simulink model "SWC_HALOUT_type"  (R2021b)
settings: Solver=FixedStepDiscrete  StartTime=0.0  StopTime=10.0  FixedStep=0.005  RelTol=1e-3
undefined symbols (not defined in the file): DIDLen_APPD, DIDLen_APPE, DIDLen_APPPedalZP, DIDLen_APSFunConfig, DIDLen_AutoLock, DIDLen_AutoWipHSpdEN, DIDLen_CALID, DIDLen_CDEODT, DIDLen_CLRDIST, DIDLen_DKCBLESta, DIDLen_DKCKey, DIDLen_DKCSta, DIDLen_DoorNFCAnchorSta, DIDLen_DRLDis, DIDLen_DynoMode, DIDLen_ECUNAME, DIDLen_FDDKCCoordXY, DIDLen_FMHTimer, DIDLen_LFLowPresThre, DIDLen_LFSensorID, DIDLen_LIDAAnchorSta, DIDLen_LRLowPresThre, DIDLen_LRSensorID, DIDLen_MILDIST, DIDLen_NUMPSATRIPSFLTMEMCLR, DIDLen_NVMPedalZP, DIDLen_OBDReq, DIDLen_ODOMETER, DIDLen_PKE, DIDLen_ProtocolId, DIDLen_PSA, DIDLen_QTYPSATRIPS, DIDLen_RFLowPresThre, DIDLen_RFSensorID, DIDLen_RRLowPresThre, DIDLen_RRSensorID, DIDLen_RUNTM, DIDLen_SensorMode, DIDLen_TestGroup, DIDLen_TireSize, DIDLen_TPMSLearnSta, DIDLen_TurnLampFLThreCurr, DIDLen_TurnLampFRThreCurr, DIDLen_TurnLampRLThreCurr, DIDLen_TurnLampRRThreCurr, DIDLen_UIDSta, DIDLen_USSConfig, DIDLen_UWBAnchorSta, DIDLen_VIN, DIDLen_VSS, DIDLen_WhlPres, DIDLen_WhlSensorBattSta, DIDLen_WhlTmp, DIDLen_WipRLSCmdCutFilter, DIDLen_WipRLSCmdHoldFilter, DIDLen_XWDMode, DIDNum_APPD, DIDNum_APPE, DIDNum_APPPedalZP, DIDNum_APSFunConfig ... (+504)
libraries: simulink x893, FVT_lib x320, hdlsllib x6, hcu_lib x5, halout x1
(part 8 of 11)

== system SWC_HALOUT_type/run_SWC_HALOUT_Tx_5ms_sys/OUTP_AFTER/DID_list/uint32Touint8Array49 ==
  In1 : Inport
  Bitwise AND1 : simulink/Logic and Bit Operations/Bitwise Operator  logicop=AND  UseBitMask=on  BitMask=bin2dec('00000000000000000000000011111111')  BitMaskRealWorld=Stored Integer
  Bitwise AND2 : simulink/Logic and Bit Operations/Bitwise Operator  logicop=AND  UseBitMask=on  BitMask=bin2dec('00000000000000001111111100000000')  BitMaskRealWorld=Stored Integer
  Bitwise AND3 : simulink/Logic and Bit Operations/Bitwise Operator  logicop=AND  UseBitMask=on  BitMask=bin2dec('00000000111111110000000000000000')  BitMaskRealWorld=Stored Integer
  Bitwise AND4 : simulink/Logic and Bit Operations/Bitwise Operator  logicop=AND  UseBitMask=on  BitMask=bin2dec('11111111000000000000000000000000')  BitMaskRealWorld=Stored Integer
  Data Type Conversion{1,3..5} (4 alike) : DataTypeConversion  OutDataTypeStr=uint8
  Data Type Conversion2 : DataTypeConversion  OutDataTypeStr=uint32
  Mux2 : Mux
  Shift Arithmetic39 : ArithShift  BitShiftNumber=8  BitShiftDirection=Right
  Shift Arithmetic40 : ArithShift  BitShiftNumber=16  BitShiftDirection=Right
  Shift Arithmetic41 : ArithShift  BitShiftNumber=24  BitShiftDirection=Right
  Out1 : Outport
  wires:
  Bitwise AND4/1 -> Shift Arithmetic41/1
  Bitwise AND1/1 -> Data Type Conversion1/1
  Shift Arithmetic40/1 -> Data Type Conversion4/1
  Shift Arithmetic41/1 -> Data Type Conversion3/1
  Mux2/1 -> Out1/1
  In1/1 -> Data Type Conversion2/1
  Bitwise AND3/1 -> Shift Arithmetic40/1
  Shift Arithmetic39/1 -> Data Type Conversion5/1
  Data Type Conversion3/1 -> Mux2/1
  Bitwise AND2/1 -> Shift Arithmetic39/1
  Data Type Conversion2/1 -> Bitwise AND4/1, Bitwise AND3/1, Bitwise AND1/1, Bitwise AND2/1
  Data Type Conversion5/1 -> Mux2/3
  Data Type Conversion4/1 -> Mux2/2
  Data Type Conversion1/1 -> Mux2/4

== system SWC_HALOUT_type/run_SWC_HALOUT_Tx_5ms_sys/OUTP_AFTER/DID_list/uint32Touint8Array5 ==
  In1 : Inport
  Bitwise AND1 : simulink/Logic and Bit Operations/Bitwise Operator  logicop=AND  UseBitMask=on  BitMask=bin2dec('00000000000000000000000011111111')  BitMaskRealWorld=Stored Integer
  Bitwise AND2 : simulink/Logic and Bit Operations/Bitwise Operator  logicop=AND  UseBitMask=on  BitMask=bin2dec('00000000000000001111111100000000')  BitMaskRealWorld=Stored Integer
  Bitwise AND3 : simulink/Logic and Bit Operations/Bitwise Operator  logicop=AND  UseBitMask=on  BitMask=bin2dec('00000000111111110000000000000000')  BitMaskRealWorld=Stored Integer
  Bitwise AND4 : simulink/Logic and Bit Operations/Bitwise Operator  logicop=AND  UseBitMask=on  BitMask=bin2dec('11111111000000000000000000000000')  BitMaskRealWorld=Stored Integer
  Data Type Conversion{1,3..5} (4 alike) : DataTypeConversion  OutDataTypeStr=uint8
  Data Type Conversion2 : DataTypeConversion  OutDataTypeStr=uint32
  Mux2 : Mux
  Shift Arithmetic39 : ArithShift  BitShiftNumber=8  BitShiftDirection=Right
  Shift Arithmetic40 : ArithShift  BitShiftNumber=16  BitShiftDirection=Right
  Shift Arithmetic41 : ArithShift  BitShiftNumber=24  BitShiftDirection=Right
  Out1 : Outport
  wires:
  Data Type Conversion1/1 -> Mux2/4
  Data Type Conversion4/1 -> Mux2/2
  Data Type Conversion5/1 -> Mux2/3
  Data Type Conversion2/1 -> Bitwise AND2/1, Bitwise AND1/1, Bitwise AND3/1, Bitwise AND4/1
  Bitwise AND2/1 -> Shift Arithmetic39/1
  Data Type Conversion3/1 -> Mux2/1
  Shift Arithmetic39/1 -> Data Type Conversion5/1
  Bitwise AND3/1 -> Shift Arithmetic40/1
  In1/1 -> Data Type Conversion2/1
  Mux2/1 -> Out1/1
  Shift Arithmetic41/1 -> Data Type Conversion3/1
  Shift Arithmetic40/1 -> Data Type Conversion4/1
  Bitwise AND1/1 -> Data Type Conversion1/1
  Bitwise AND4/1 -> Shift Arithmetic41/1

== system SWC_HALOUT_type/run_SWC_HALOUT_Tx_5ms_sys/OUTP_AFTER/DID_list/uint32Touint8Array50 ==
  In1 : Inport
  Bitwise AND1 : simulink/Logic and Bit Operations/Bitwise Operator  logicop=AND  UseBitMask=on  BitMask=bin2dec('00000000000000000000000011111111')  BitMaskRealWorld=Stored Integer
  Bitwise AND2 : simulink/Logic and Bit Operations/Bitwise Operator  logicop=AND  UseBitMask=on  BitMask=bin2dec('00000000000000001111111100000000')  BitMaskRealWorld=Stored Integer
  Bitwise AND3 : simulink/Logic and Bit Operations/Bitwise Operator  logicop=AND  UseBitMask=on  BitMask=bin2dec('00000000111111110000000000000000')  BitMaskRealWorld=Stored Integer
  Bitwise AND4 : simulink/Logic and Bit Operations/Bitwise Operator  logicop=AND  UseBitMask=on  BitMask=bin2dec('11111111000000000000000000000000')  BitMaskRealWorld=Stored Integer
  Data Type Conversion{1,3..5} (4 alike) : DataTypeConversion  OutDataTypeStr=uint8
  Data Type Conversion2 : DataTypeConversion  OutDataTypeStr=uint32
  Mux2 : Mux
  Shift Arithmetic39 : ArithShift  BitShiftNumber=8  BitShiftDirection=Right
  Shift Arithmetic40 : ArithShift  BitShiftNumber=16  BitShiftDirection=Right
  Shift Arithmetic41 : ArithShift  BitShiftNumber=24  BitShiftDirection=Right
  Out1 : Outport
  wires:
  Data Type Conversion1/1 -> Mux2/4
  Data Type Conversion4/1 -> Mux2/2
  Data Type Conversion5/1 -> Mux2/3
  Data Type Conversion2/1 -> Bitwise AND2/1, Bitwise AND1/1, Bitwise AND3/1, Bitwise AND4/1
  Bitwise AND2/1 -> Shift Arithmetic39/1
  Data Type Conversion3/1 -> Mux2/1
  Shift Arithmetic39/1 -> Data Type Conversion5/1
  Bitwise AND3/1 -> Shift Arithmetic40/1
  In1/1 -> Data Type Conversion2/1
  Mux2/1 -> Out1/1
  Shift Arithmetic41/1 -> Data Type Conversion3/1
  Shift Arithmetic40/1 -> Data Type Conversion4/1
  Bitwise AND1/1 -> Data Type Conversion1/1
  Bitwise AND4/1 -> Shift Arithmetic41/1

== system SWC_HALOUT_type/run_SWC_HALOUT_Tx_5ms_sys/OUTP_AFTER/DID_list/uint32Touint8Array51 ==
  In1 : Inport
  Bitwise AND1 : simulink/Logic and Bit Operations/Bitwise Operator  logicop=AND  UseBitMask=on  BitMask=bin2dec('00000000000000000000000011111111')  BitMaskRealWorld=Stored Integer
  Bitwise AND2 : simulink/Logic and Bit Operations/Bitwise Operator  logicop=AND  UseBitMask=on  BitMask=bin2dec('00000000000000001111111100000000')  BitMaskRealWorld=Stored Integer
  Bitwise AND3 : simulink/Logic and Bit Operations/Bitwise Operator  logicop=AND  UseBitMask=on  BitMask=bin2dec('00000000111111110000000000000000')  BitMaskRealWorld=Stored Integer
  Bitwise AND4 : simulink/Logic and Bit Operations/Bitwise Operator  logicop=AND  UseBitMask=on  BitMask=bin2dec('11111111000000000000000000000000')  BitMaskRealWorld=Stored Integer
  Data Type Conversion{1,3..5} (4 alike) : DataTypeConversion  OutDataTypeStr=uint8
  Data Type Conversion2 : DataTypeConversion  OutDataTypeStr=uint32
  Mux2 : Mux
  Shift Arithmetic39 : ArithShift  BitShiftNumber=8  BitShiftDirection=Right
  Shift Arithmetic40 : ArithShift  BitShiftNumber=16  BitShiftDirection=Right
  Shift Arithmetic41 : ArithShift  BitShiftNumber=24  BitShiftDirection=Right
  Out1 : Outport
  wires:
  Bitwise AND4/1 -> Shift Arithmetic41/1
  Bitwise AND1/1 -> Data Type Conversion1/1
  Shift Arithmetic40/1 -> Data Type Conversion4/1
  Shift Arithmetic41/1 -> Data Type Conversion3/1
  Mux2/1 -> Out1/1
  In1/1 -> Data Type Conversion2/1
  Bitwise AND3/1 -> Shift Arithmetic40/1
  Shift Arithmetic39/1 -> Data Type Conversion5/1
  Data Type Conversion3/1 -> Mux2/1
  Bitwise AND2/1 -> Shift Arithmetic39/1
  Data Type Conversion2/1 -> Bitwise AND4/1, Bitwise AND3/1, Bitwise AND1/1, Bitwise AND2/1
  Data Type Conversion5/1 -> Mux2/3
  Data Type Conversion4/1 -> Mux2/2
  Data Type Conversion1/1 -> Mux2/4

== system SWC_HALOUT_type/run_SWC_HALOUT_Tx_5ms_sys/OUTP_AFTER/DID_list/uint32Touint8Array52 ==
  In1 : Inport
  Bitwise AND1 : simulink/Logic and Bit Operations/Bitwise Operator  logicop=AND  UseBitMask=on  BitMask=bin2dec('00000000000000000000000011111111')  BitMaskRealWorld=Stored Integer
  Bitwise AND2 : simulink/Logic and Bit Operations/Bitwise Operator  logicop=AND  UseBitMask=on  BitMask=bin2dec('00000000000000001111111100000000')  BitMaskRealWorld=Stored Integer
  Bitwise AND3 : simulink/Logic and Bit Operations/Bitwise Operator  logicop=AND  UseBitMask=on  BitMask=bin2dec('00000000111111110000000000000000')  BitMaskRealWorld=Stored Integer
  Bitwise AND4 : simulink/Logic and Bit Operations/Bitwise Operator  logicop=AND  UseBitMask=on  BitMask=bin2dec('11111111000000000000000000000000')  BitMaskRealWorld=Stored Integer
  Data Type Conversion{1,3..5} (4 alike) : DataTypeConversion  OutDataTypeStr=uint8
  Data Type Conversion2 : DataTypeConversion  OutDataTypeStr=uint32
  Mux2 : Mux
  Shift Arithmetic39 : ArithShift  BitShiftNumber=8  BitShiftDirection=Right
  Shift Arithmetic40 : ArithShift  BitShiftNumber=16  BitShiftDirection=Right
  Shift Arithmetic41 : ArithShift  BitShiftNumber=24  BitShiftDirection=Right
  Out1 : Outport
  wires:
  Data Type Conversion1/1 -> Mux2/4
  Data Type Conversion4/1 -> Mux2/2
  Data Type Conversion5/1 -> Mux2/3
  Data Type Conversion2/1 -> Bitwise AND2/1, Bitwise AND1/1, Bitwise AND3/1, Bitwise AND4/1
  Bitwise AND2/1 -> Shift Arithmetic39/1
  Data Type Conversion3/1 -> Mux2/1
  Shift Arithmetic39/1 -> Data Type Conversion5/1
  Bitwise AND3/1 -> Shift Arithmetic40/1
  In1/1 -> Data Type Conversion2/1
  Mux2/1 -> Out1/1
  Shift Arithmetic41/1 -> Data Type Conversion3/1
  Shift Arithmetic40/1 -> Data Type Conversion4/1
  Bitwise AND1/1 -> Data Type Conversion1/1
  Bitwise AND4/1 -> Shift Arithmetic41/1

== system SWC_HALOUT_type/run_SWC_HALOUT_Tx_5ms_sys/OUTP_AFTER/DID_list/uint32Touint8Array53 ==
  In1 : Inport
  Bitwise AND1 : simulink/Logic and Bit Operations/Bitwise Operator  logicop=AND  UseBitMask=on  BitMask=bin2dec('00000000000000000000000011111111')  BitMaskRealWorld=Stored Integer
  Bitwise AND2 : simulink/Logic and Bit Operations/Bitwise Operator  logicop=AND  UseBitMask=on  BitMask=bin2dec('00000000000000001111111100000000')  BitMaskRealWorld=Stored Integer
  Bitwise AND3 : simulink/Logic and Bit Operations/Bitwise Operator  logicop=AND  UseBitMask=on  BitMask=bin2dec('00000000111111110000000000000000')  BitMaskRealWorld=Stored Integer
  Bitwise AND4 : simulink/Logic and Bit Operations/Bitwise Operator  logicop=AND  UseBitMask=on  BitMask=bin2dec('11111111000000000000000000000000')  BitMaskRealWorld=Stored Integer
  Data Type Conversion{1,3..5} (4 alike) : DataTypeConversion  OutDataTypeStr=uint8
  Data Type Conversion2 : DataTypeConversion  OutDataTypeStr=uint32
  Mux2 : Mux
  Shift Arithmetic39 : ArithShift  BitShiftNumber=8  BitShiftDirection=Right
  Shift Arithmetic40 : ArithShift  BitShiftNumber=16  BitShiftDirection=Right
  Shift Arithmetic41 : ArithShift  BitShiftNumber=24  BitShiftDirection=Right
  Out1 : Outport
  wires:
  Data Type Conversion1/1 -> Mux2/4
  Data Type Conversion4/1 -> Mux2/2
  Data Type Conversion5/1 -> Mux2/3
  Data Type Conversion2/1 -> Bitwise AND2/1, Bitwise AND1/1, Bitwise AND3/1, Bitwise AND4/1
  Bitwise AND2/1 -> Shift Arithmetic39/1
  Data Type Conversion3/1 -> Mux2/1
  Shift Arithmetic39/1 -> Data Type Conversion5/1
  Bitwise AND3/1 -> Shift Arithmetic40/1
  In1/1 -> Data Type Conversion2/1
  Mux2/1 -> Out1/1
  Shift Arithmetic41/1 -> Data Type Conversion3/1
  Shift Arithmetic40/1 -> Data Type Conversion4/1
  Bitwise AND1/1 -> Data Type Conversion1/1
  Bitwise AND4/1 -> Shift Arithmetic41/1

== system SWC_HALOUT_type/run_SWC_HALOUT_Tx_5ms_sys/OUTP_AFTER/DID_list/uint32Touint8Array54 ==
  In1 : Inport
  Bitwise AND1 : simulink/Logic and Bit Operations/Bitwise Operator  logicop=AND  UseBitMask=on  BitMask=bin2dec('00000000000000000000000011111111')  BitMaskRealWorld=Stored Integer
  Bitwise AND2 : simulink/Logic and Bit Operations/Bitwise Operator  logicop=AND  UseBitMask=on  BitMask=bin2dec('00000000000000001111111100000000')  BitMaskRealWorld=Stored Integer
  Bitwise AND3 : simulink/Logic and Bit Operations/Bitwise Operator  logicop=AND  UseBitMask=on  BitMask=bin2dec('00000000111111110000000000000000')  BitMaskRealWorld=Stored Integer
  Bitwise AND4 : simulink/Logic and Bit Operations/Bitwise Operator  logicop=AND  UseBitMask=on  BitMask=bin2dec('11111111000000000000000000000000')  BitMaskRealWorld=Stored Integer
  Data Type Conversion{1,3..5} (4 alike) : DataTypeConversion  OutDataTypeStr=uint8
  Data Type Conversion2 : DataTypeConversion  OutDataTypeStr=uint32
  Mux2 : Mux
  Shift Arithmetic39 : ArithShift  BitShiftNumber=8  BitShiftDirection=Right
  Shift Arithmetic40 : ArithShift  BitShiftNumber=16  BitShiftDirection=Right
  Shift Arithmetic41 : ArithShift  BitShiftNumber=24  BitShiftDirection=Right
  Out1 : Outport
  wires:
  Bitwise AND4/1 -> Shift Arithmetic41/1
  Bitwise AND1/1 -> Data Type Conversion1/1
  Shift Arithmetic40/1 -> Data Type Conversion4/1
  Shift Arithmetic41/1 -> Data Type Conversion3/1
  Mux2/1 -> Out1/1
  In1/1 -> Data Type Conversion2/1
  Bitwise AND3/1 -> Shift Arithmetic40/1
  Shift Arithmetic39/1 -> Data Type Conversion5/1
  Data Type Conversion3/1 -> Mux2/1
  Bitwise AND2/1 -> Shift Arithmetic39/1
  Data Type Conversion2/1 -> Bitwise AND4/1, Bitwise AND3/1, Bitwise AND1/1, Bitwise AND2/1
  Data Type Conversion5/1 -> Mux2/3
  Data Type Conversion4/1 -> Mux2/2
  Data Type Conversion1/1 -> Mux2/4

== system SWC_HALOUT_type/run_SWC_HALOUT_Tx_5ms_sys/OUTP_AFTER/DID_list/uint32Touint8Array55 ==
  In1 : Inport
  Bitwise AND1 : simulink/Logic and Bit Operations/Bitwise Operator  logicop=AND  UseBitMask=on  BitMask=bin2dec('00000000000000000000000011111111')  BitMaskRealWorld=Stored Integer
  Bitwise AND2 : simulink/Logic and Bit Operations/Bitwise Operator  logicop=AND  UseBitMask=on  BitMask=bin2dec('00000000000000001111111100000000')  BitMaskRealWorld=Stored Integer
  Bitwise AND3 : simulink/Logic and Bit Operations/Bitwise Operator  logicop=AND  UseBitMask=on  BitMask=bin2dec('00000000111111110000000000000000')  BitMaskRealWorld=Stored Integer
  Bitwise AND4 : simulink/Logic and Bit Operations/Bitwise Operator  logicop=AND  UseBitMask=on  BitMask=bin2dec('11111111000000000000000000000000')  BitMaskRealWorld=Stored Integer
  Data Type Conversion{1,3..5} (4 alike) : DataTypeConversion  OutDataTypeStr=uint8
  Data Type Conversion2 : DataTypeConversion  OutDataTypeStr=uint32
  Mux2 : Mux
  Shift Arithmetic39 : ArithShift  BitShiftNumber=8  BitShiftDirection=Right
  Shift Arithmetic40 : ArithShift  BitShiftNumber=16  BitShiftDirection=Right
  Shift Arithmetic41 : ArithShift  BitShiftNumber=24  BitShiftDirection=Right
  Out1 : Outport
  wires:
  Data Type Conversion1/1 -> Mux2/4
  Data Type Conversion4/1 -> Mux2/2
  Data Type Conversion5/1 -> Mux2/3
  Data Type Conversion2/1 -> Bitwise AND2/1, Bitwise AND1/1, Bitwise AND3/1, Bitwise AND4/1
  Bitwise AND2/1 -> Shift Arithmetic39/1
  Data Type Conversion3/1 -> Mux2/1
  Shift Arithmetic39/1 -> Data Type Conversion5/1
  Bitwise AND3/1 -> Shift Arithmetic40/1
  In1/1 -> Data Type Conversion2/1
  Mux2/1 -> Out1/1
  Shift Arithmetic41/1 -> Data Type Conversion3/1
  Shift Arithmetic40/1 -> Data Type Conversion4/1
  Bitwise AND1/1 -> Data Type Conversion1/1
  Bitwise AND4/1 -> Shift Arithmetic41/1

== system SWC_HALOUT_type/run_SWC_HALOUT_Tx_5ms_sys/OUTP_AFTER/DID_list/uint32Touint8Array56 ==
  In1 : Inport
  Bitwise AND1 : simulink/Logic and Bit Operations/Bitwise Operator  logicop=AND  UseBitMask=on  BitMask=bin2dec('00000000000000000000000011111111')  BitMaskRealWorld=Stored Integer
  Bitwise AND2 : simulink/Logic and Bit Operations/Bitwise Operator  logicop=AND  UseBitMask=on  BitMask=bin2dec('00000000000000001111111100000000')  BitMaskRealWorld=Stored Integer
  Bitwise AND3 : simulink/Logic and Bit Operations/Bitwise Operator  logicop=AND  UseBitMask=on  BitMask=bin2dec('00000000111111110000000000000000')  BitMaskRealWorld=Stored Integer
  Bitwise AND4 : simulink/Logic and Bit Operations/Bitwise Operator  logicop=AND  UseBitMask=on  BitMask=bin2dec('11111111000000000000000000000000')  BitMaskRealWorld=Stored Integer
  Data Type Conversion{1,3..5} (4 alike) : DataTypeConversion  OutDataTypeStr=uint8
  Data Type Conversion2 : DataTypeConversion  OutDataTypeStr=uint32
  Mux2 : Mux
  Shift Arithmetic39 : ArithShift  BitShiftNumber=8  BitShiftDirection=Right
  Shift Arithmetic40 : ArithShift  BitShiftNumber=16  BitShiftDirection=Right
  Shift Arithmetic41 : ArithShift  BitShiftNumber=24  BitShiftDirection=Right
  Out1 : Outport
  wires:
  Bitwise AND4/1 -> Shift Arithmetic41/1
  Bitwise AND1/1 -> Data Type Conversion1/1
  Shift Arithmetic40/1 -> Data Type Conversion4/1
  Shift Arithmetic41/1 -> Data Type Conversion3/1
  Mux2/1 -> Out1/1
  In1/1 -> Data Type Conversion2/1
  Bitwise AND3/1 -> Shift Arithmetic40/1
  Shift Arithmetic39/1 -> Data Type Conversion5/1
  Data Type Conversion3/1 -> Mux2/1
  Bitwise AND2/1 -> Shift Arithmetic39/1
  Data Type Conversion2/1 -> Bitwise AND4/1, Bitwise AND3/1, Bitwise AND1/1, Bitwise AND2/1
  Data Type Conversion5/1 -> Mux2/3
  Data Type Conversion4/1 -> Mux2/2
  Data Type Conversion1/1 -> Mux2/4

== system SWC_HALOUT_type/run_SWC_HALOUT_Tx_5ms_sys/OUTP_AFTER/DID_list/uint32Touint8Array57 ==
  In1 : Inport
  Bitwise AND1 : simulink/Logic and Bit Operations/Bitwise Operator  logicop=AND  UseBitMask=on  BitMask=bin2dec('00000000000000000000000011111111')  BitMaskRealWorld=Stored Integer
  Bitwise AND2 : simulink/Logic and Bit Operations/Bitwise Operator  logicop=AND  UseBitMask=on  BitMask=bin2dec('00000000000000001111111100000000')  BitMaskRealWorld=Stored Integer
  Bitwise AND3 : simulink/Logic and Bit Operations/Bitwise Operator  logicop=AND  UseBitMask=on  BitMask=bin2dec('00000000111111110000000000000000')  BitMaskRealWorld=Stored Integer
  Bitwise AND4 : simulink/Logic and Bit Operations/Bitwise Operator  logicop=AND  UseBitMask=on  BitMask=bin2dec('11111111000000000000000000000000')  BitMaskRealWorld=Stored Integer
  Data Type Conversion{1,3..5} (4 alike) : DataTypeConversion  OutDataTypeStr=uint8
  Data Type Conversion2 : DataTypeConversion  OutDataTypeStr=uint32
  Mux2 : Mux
  Shift Arithmetic39 : ArithShift  BitShiftNumber=8  BitShiftDirection=Right
  Shift Arithmetic40 : ArithShift  BitShiftNumber=16  BitShiftDirection=Right
  Shift Arithmetic41 : ArithShift  BitShiftNumber=24  BitShiftDirection=Right
  Out1 : Outport
  wires:
  Bitwise AND4/1 -> Shift Arithmetic41/1
  Bitwise AND1/1 -> Data Type Conversion1/1
  Shift Arithmetic40/1 -> Data Type Conversion4/1
  Shift Arithmetic41/1 -> Data Type Conversion3/1
  Mux2/1 -> Out1/1
  In1/1 -> Data Type Conversion2/1
  Bitwise AND3/1 -> Shift Arithmetic40/1
  Shift Arithmetic39/1 -> Data Type Conversion5/1
  Data Type Conversion3/1 -> Mux2/1
  Bitwise AND2/1 -> Shift Arithmetic39/1
  Data Type Conversion2/1 -> Bitwise AND4/1, Bitwise AND3/1, Bitwise AND1/1, Bitwise AND2/1
  Data Type Conversion5/1 -> Mux2/3
  Data Type Conversion4/1 -> Mux2/2
  Data Type Conversion1/1 -> Mux2/4

== system SWC_HALOUT_type/run_SWC_HALOUT_Tx_5ms_sys/OUTP_AFTER/DID_list/uint32Touint8Array58 ==
  In1 : Inport
  Bitwise AND1 : simulink/Logic and Bit Operations/Bitwise Operator  logicop=AND  UseBitMask=on  BitMask=bin2dec('00000000000000000000000011111111')  BitMaskRealWorld=Stored Integer
  Bitwise AND2 : simulink/Logic and Bit Operations/Bitwise Operator  logicop=AND  UseBitMask=on  BitMask=bin2dec('00000000000000001111111100000000')  BitMaskRealWorld=Stored Integer
  Bitwise AND3 : simulink/Logic and Bit Operations/Bitwise Operator  logicop=AND  UseBitMask=on  BitMask=bin2dec('00000000111111110000000000000000')  BitMaskRealWorld=Stored Integer
  Bitwise AND4 : simulink/Logic and Bit Operations/Bitwise Operator  logicop=AND  UseBitMask=on  BitMask=bin2dec('11111111000000000000000000000000')  BitMaskRealWorld=Stored Integer
  Data Type Conversion{1,3..5} (4 alike) : DataTypeConversion  OutDataTypeStr=uint8
  Data Type Conversion2 : DataTypeConversion  OutDataTypeStr=uint32
  Mux2 : Mux
  Shift Arithmetic39 : ArithShift  BitShiftNumber=8  BitShiftDirection=Right
  Shift Arithmetic40 : ArithShift  BitShiftNumber=16  BitShiftDirection=Right
  Shift Arithmetic41 : ArithShift  BitShiftNumber=24  BitShiftDirection=Right
  Out1 : Outport
  wires:
  Data Type Conversion1/1 -> Mux2/4
  Data Type Conversion4/1 -> Mux2/2
  Data Type Conversion5/1 -> Mux2/3
  Data Type Conversion2/1 -> Bitwise AND2/1, Bitwise AND1/1, Bitwise AND3/1, Bitwise AND4/1
  Bitwise AND2/1 -> Shift Arithmetic39/1
  Data Type Conversion3/1 -> Mux2/1
  Shift Arithmetic39/1 -> Data Type Conversion5/1
  Bitwise AND3/1 -> Shift Arithmetic40/1
  In1/1 -> Data Type Conversion2/1
  Mux2/1 -> Out1/1
  Shift Arithmetic41/1 -> Data Type Conversion3/1
  Shift Arithmetic40/1 -> Data Type Conversion4/1
  Bitwise AND1/1 -> Data Type Conversion1/1
  Bitwise AND4/1 -> Shift Arithmetic41/1

== system SWC_HALOUT_type/run_SWC_HALOUT_Tx_5ms_sys/OUTP_AFTER/DID_list/uint32Touint8Array59 ==
  In1 : Inport
  Bitwise AND1 : simulink/Logic and Bit Operations/Bitwise Operator  logicop=AND  UseBitMask=on  BitMask=bin2dec('00000000000000000000000011111111')  BitMaskRealWorld=Stored Integer
  Bitwise AND2 : simulink/Logic and Bit Operations/Bitwise Operator  logicop=AND  UseBitMask=on  BitMask=bin2dec('00000000000000001111111100000000')  BitMaskRealWorld=Stored Integer
  Bitwise AND3 : simulink/Logic and Bit Operations/Bitwise Operator  logicop=AND  UseBitMask=on  BitMask=bin2dec('00000000111111110000000000000000')  BitMaskRealWorld=Stored Integer
  Bitwise AND4 : simulink/Logic and Bit Operations/Bitwise Operator  logicop=AND  UseBitMask=on  BitMask=bin2dec('11111111000000000000000000000000')  BitMaskRealWorld=Stored Integer
  Data Type Conversion{1,3..5} (4 alike) : DataTypeConversion  OutDataTypeStr=uint8
  Data Type Conversion2 : DataTypeConversion  OutDataTypeStr=uint32
  Mux2 : Mux
  Shift Arithmetic39 : ArithShift  BitShiftNumber=8  BitShiftDirection=Right
  Shift Arithmetic40 : ArithShift  BitShiftNumber=16  BitShiftDirection=Right
  Shift Arithmetic41 : ArithShift  BitShiftNumber=24  BitShiftDirection=Right
  Out1 : Outport
  wires:
  Bitwise AND4/1 -> Shift Arithmetic41/1
  Bitwise AND1/1 -> Data Type Conversion1/1
  Shift Arithmetic40/1 -> Data Type Conversion4/1
  Shift Arithmetic41/1 -> Data Type Conversion3/1
  Mux2/1 -> Out1/1
  In1/1 -> Data Type Conversion2/1
  Bitwise AND3/1 -> Shift Arithmetic40/1
  Shift Arithmetic39/1 -> Data Type Conversion5/1
  Data Type Conversion3/1 -> Mux2/1
  Bitwise AND2/1 -> Shift Arithmetic39/1
  Data Type Conversion2/1 -> Bitwise AND4/1, Bitwise AND3/1, Bitwise AND1/1, Bitwise AND2/1
  Data Type Conversion5/1 -> Mux2/3
  Data Type Conversion4/1 -> Mux2/2
  Data Type Conversion1/1 -> Mux2/4

== system SWC_HALOUT_type/run_SWC_HALOUT_Tx_5ms_sys/OUTP_AFTER/DID_list/uint32Touint8Array6 ==
  In1 : Inport
  Bitwise AND1 : simulink/Logic and Bit Operations/Bitwise Operator  logicop=AND  UseBitMask=on  BitMask=bin2dec('00000000000000000000000011111111')  BitMaskRealWorld=Stored Integer
  Bitwise AND2 : simulink/Logic and Bit Operations/Bitwise Operator  logicop=AND  UseBitMask=on  BitMask=bin2dec('00000000000000001111111100000000')  BitMaskRealWorld=Stored Integer
  Bitwise AND3 : simulink/Logic and Bit Operations/Bitwise Operator  logicop=AND  UseBitMask=on  BitMask=bin2dec('00000000111111110000000000000000')  BitMaskRealWorld=Stored Integer
  Bitwise AND4 : simulink/Logic and Bit Operations/Bitwise Operator  logicop=AND  UseBitMask=on  BitMask=bin2dec('11111111000000000000000000000000')  BitMaskRealWorld=Stored Integer
  Data Type Conversion{1,3..5} (4 alike) : DataTypeConversion  OutDataTypeStr=uint8
  Data Type Conversion2 : DataTypeConversion  OutDataTypeStr=uint32
  Mux2 : Mux
  Shift Arithmetic39 : ArithShift  BitShiftNumber=8  BitShiftDirection=Right
  Shift Arithmetic40 : ArithShift  BitShiftNumber=16  BitShiftDirection=Right
  Shift Arithmetic41 : ArithShift  BitShiftNumber=24  BitShiftDirection=Right
  Out1 : Outport
  wires:
  Bitwise AND4/1 -> Shift Arithmetic41/1
  Bitwise AND1/1 -> Data Type Conversion1/1
  Shift Arithmetic40/1 -> Data Type Conversion4/1
  Shift Arithmetic41/1 -> Data Type Conversion3/1
  Mux2/1 -> Out1/1
  In1/1 -> Data Type Conversion2/1
  Bitwise AND3/1 -> Shift Arithmetic40/1
  Shift Arithmetic39/1 -> Data Type Conversion5/1
  Data Type Conversion3/1 -> Mux2/1
  Bitwise AND2/1 -> Shift Arithmetic39/1
  Data Type Conversion2/1 -> Bitwise AND4/1, Bitwise AND3/1, Bitwise AND1/1, Bitwise AND2/1
  Data Type Conversion5/1 -> Mux2/3
  Data Type Conversion4/1 -> Mux2/2
  Data Type Conversion1/1 -> Mux2/4

== system SWC_HALOUT_type/run_SWC_HALOUT_Tx_5ms_sys/OUTP_AFTER/DID_list/uint32Touint8Array60 ==
  In1 : Inport
  Bitwise AND1 : simulink/Logic and Bit Operations/Bitwise Operator  logicop=AND  UseBitMask=on  BitMask=bin2dec('00000000000000000000000011111111')  BitMaskRealWorld=Stored Integer
  Bitwise AND2 : simulink/Logic and Bit Operations/Bitwise Operator  logicop=AND  UseBitMask=on  BitMask=bin2dec('00000000000000001111111100000000')  BitMaskRealWorld=Stored Integer
  Bitwise AND3 : simulink/Logic and Bit Operations/Bitwise Operator  logicop=AND  UseBitMask=on  BitMask=bin2dec('00000000111111110000000000000000')  BitMaskRealWorld=Stored Integer
  Bitwise AND4 : simulink/Logic and Bit Operations/Bitwise Operator  logicop=AND  UseBitMask=on  BitMask=bin2dec('11111111000000000000000000000000')  BitMaskRealWorld=Stored Integer
  Data Type Conversion{1,3..5} (4 alike) : DataTypeConversion  OutDataTypeStr=uint8
  Data Type Conversion2 : DataTypeConversion  OutDataTypeStr=uint32
  Mux2 : Mux
  Shift Arithmetic39 : ArithShift  BitShiftNumber=8  BitShiftDirection=Right
  Shift Arithmetic40 : ArithShift  BitShiftNumber=16  BitShiftDirection=Right
  Shift Arithmetic41 : ArithShift  BitShiftNumber=24  BitShiftDirection=Right
  Out1 : Outport
  wires:
  Data Type Conversion1/1 -> Mux2/4
  Data Type Conversion4/1 -> Mux2/2
  Data Type Conversion5/1 -> Mux2/3
  Data Type Conversion2/1 -> Bitwise AND2/1, Bitwise AND1/1, Bitwise AND3/1, Bitwise AND4/1
  Bitwise AND2/1 -> Shift Arithmetic39/1
  Data Type Conversion3/1 -> Mux2/1
  Shift Arithmetic39/1 -> Data Type Conversion5/1
  Bitwise AND3/1 -> Shift Arithmetic40/1
  In1/1 -> Data Type Conversion2/1
  Mux2/1 -> Out1/1
  Shift Arithmetic41/1 -> Data Type Conversion3/1
  Shift Arithmetic40/1 -> Data Type Conversion4/1
  Bitwise AND1/1 -> Data Type Conversion1/1
  Bitwise AND4/1 -> Shift Arithmetic41/1

== system SWC_HALOUT_type/run_SWC_HALOUT_Tx_5ms_sys/OUTP_AFTER/DID_list/uint32Touint8Array61 ==
  In1 : Inport
  Bitwise AND1 : simulink/Logic and Bit Operations/Bitwise Operator  logicop=AND  UseBitMask=on  BitMask=bin2dec('00000000000000000000000011111111')  BitMaskRealWorld=Stored Integer
  Bitwise AND2 : simulink/Logic and Bit Operations/Bitwise Operator  logicop=AND  UseBitMask=on  BitMask=bin2dec('00000000000000001111111100000000')  BitMaskRealWorld=Stored Integer
  Bitwise AND3 : simulink/Logic and Bit Operations/Bitwise Operator  logicop=AND  UseBitMask=on  BitMask=bin2dec('00000000111111110000000000000000')  BitMaskRealWorld=Stored Integer
  Bitwise AND4 : simulink/Logic and Bit Operations/Bitwise Operator  logicop=AND  UseBitMask=on  BitMask=bin2dec('11111111000000000000000000000000')  BitMaskRealWorld=Stored Integer
  Data Type Conversion{1,3..5} (4 alike) : DataTypeConversion  OutDataTypeStr=uint8
  Data Type Conversion2 : DataTypeConversion  OutDataTypeStr=uint32
  Mux2 : Mux
  Shift Arithmetic39 : ArithShift  BitShiftNumber=8  BitShiftDirection=Right
  Shift Arithmetic40 : ArithShift  BitShiftNumber=16  BitShiftDirection=Right
  Shift Arithmetic41 : ArithShift  BitShiftNumber=24  BitShiftDirection=Right
  Out1 : Outport
  wires:
  Data Type Conversion1/1 -> Mux2/4
  Data Type Conversion4/1 -> Mux2/2
  Data Type Conversion5/1 -> Mux2/3
  Data Type Conversion2/1 -> Bitwise AND2/1, Bitwise AND1/1, Bitwise AND3/1, Bitwise AND4/1
  Bitwise AND2/1 -> Shift Arithmetic39/1
  Data Type Conversion3/1 -> Mux2/1
  Shift Arithmetic39/1 -> Data Type Conversion5/1
  Bitwise AND3/1 -> Shift Arithmetic40/1
  In1/1 -> Data Type Conversion2/1
  Mux2/1 -> Out1/1
  Shift Arithmetic41/1 -> Data Type Conversion3/1
  Shift Arithmetic40/1 -> Data Type Conversion4/1
  Bitwise AND1/1 -> Data Type Conversion1/1
  Bitwise AND4/1 -> Shift Arithmetic41/1

== system SWC_HALOUT_type/run_SWC_HALOUT_Tx_5ms_sys/OUTP_AFTER/DID_list/uint32Touint8Array62 ==
  In1 : Inport
  Bitwise AND1 : simulink/Logic and Bit Operations/Bitwise Operator  logicop=AND  UseBitMask=on  BitMask=bin2dec('00000000000000000000000011111111')  BitMaskRealWorld=Stored Integer
  Bitwise AND2 : simulink/Logic and Bit Operations/Bitwise Operator  logicop=AND  UseBitMask=on  BitMask=bin2dec('00000000000000001111111100000000')  BitMaskRealWorld=Stored Integer
  Bitwise AND3 : simulink/Logic and Bit Operations/Bitwise Operator  logicop=AND  UseBitMask=on  BitMask=bin2dec('00000000111111110000000000000000')  BitMaskRealWorld=Stored Integer
  Bitwise AND4 : simulink/Logic and Bit Operations/Bitwise Operator  logicop=AND  UseBitMask=on  BitMask=bin2dec('11111111000000000000000000000000')  BitMaskRealWorld=Stored Integer
  Data Type Conversion{1,3..5} (4 alike) : DataTypeConversion  OutDataTypeStr=uint8
  Data Type Conversion2 : DataTypeConversion  OutDataTypeStr=uint32
  Mux2 : Mux
  Shift Arithmetic39 : ArithShift  BitShiftNumber=8  BitShiftDirection=Right
  Shift Arithmetic40 : ArithShift  BitShiftNumber=16  BitShiftDirection=Right
  Shift Arithmetic41 : ArithShift  BitShiftNumber=24  BitShiftDirection=Right
  Out1 : Outport
  wires:
  Bitwise AND4/1 -> Shift Arithmetic41/1
  Bitwise AND1/1 -> Data Type Conversion1/1
  Shift Arithmetic40/1 -> Data Type Conversion4/1
  Shift Arithmetic41/1 -> Data Type Conversion3/1
  Mux2/1 -> Out1/1
  In1/1 -> Data Type Conversion2/1
  Bitwise AND3/1 -> Shift Arithmetic40/1
  Shift Arithmetic39/1 -> Data Type Conversion5/1
  Data Type Conversion3/1 -> Mux2/1
  Bitwise AND2/1 -> Shift Arithmetic39/1
  Data Type Conversion2/1 -> Bitwise AND4/1, Bitwise AND3/1, Bitwise AND1/1, Bitwise AND2/1
  Data Type Conversion5/1 -> Mux2/3
  Data Type Conversion4/1 -> Mux2/2
  Data Type Conversion1/1 -> Mux2/4

== system SWC_HALOUT_type/run_SWC_HALOUT_Tx_5ms_sys/OUTP_AFTER/DID_list/uint32Touint8Array63 ==
  In1 : Inport
  Bitwise AND1 : simulink/Logic and Bit Operations/Bitwise Operator  logicop=AND  UseBitMask=on  BitMask=bin2dec('00000000000000000000000011111111')  BitMaskRealWorld=Stored Integer
  Bitwise AND2 : simulink/Logic and Bit Operations/Bitwise Operator  logicop=AND  UseBitMask=on  BitMask=bin2dec('00000000000000001111111100000000')  BitMaskRealWorld=Stored Integer
  Bitwise AND3 : simulink/Logic and Bit Operations/Bitwise Operator  logicop=AND  UseBitMask=on  BitMask=bin2dec('00000000111111110000000000000000')  BitMaskRealWorld=Stored Integer
  Bitwise AND4 : simulink/Logic and Bit Operations/Bitwise Operator  logicop=AND  UseBitMask=on  BitMask=bin2dec('11111111000000000000000000000000')  BitMaskRealWorld=Stored Integer
  Data Type Conversion{1,3..5} (4 alike) : DataTypeConversion  OutDataTypeStr=uint8
  Data Type Conversion2 : DataTypeConversion  OutDataTypeStr=uint32
  Mux2 : Mux
  Shift Arithmetic39 : ArithShift  BitShiftNumber=8  BitShiftDirection=Right
  Shift Arithmetic40 : ArithShift  BitShiftNumber=16  BitShiftDirection=Right
  Shift Arithmetic41 : ArithShift  BitShiftNumber=24  BitShiftDirection=Right
  Out1 : Outport
  wires:
  Bitwise AND4/1 -> Shift Arithmetic41/1
  Bitwise AND1/1 -> Data Type Conversion1/1
  Shift Arithmetic40/1 -> Data Type Conversion4/1
  Shift Arithmetic41/1 -> Data Type Conversion3/1
  Mux2/1 -> Out1/1
  In1/1 -> Data Type Conversion2/1
  Bitwise AND3/1 -> Shift Arithmetic40/1
  Shift Arithmetic39/1 -> Data Type Conversion5/1
  Data Type Conversion3/1 -> Mux2/1
  Bitwise AND2/1 -> Shift Arithmetic39/1
  Data Type Conversion2/1 -> Bitwise AND4/1, Bitwise AND3/1, Bitwise AND1/1, Bitwise AND2/1
  Data Type Conversion5/1 -> Mux2/3
  Data Type Conversion4/1 -> Mux2/2
  Data Type Conversion1/1 -> Mux2/4

== system SWC_HALOUT_type/run_SWC_HALOUT_Tx_5ms_sys/OUTP_AFTER/DID_list/uint32Touint8Array64 ==
  In1 : Inport
  Bitwise AND1 : simulink/Logic and Bit Operations/Bitwise Operator  logicop=AND  UseBitMask=on  BitMask=bin2dec('00000000000000000000000011111111')  BitMaskRealWorld=Stored Integer
  Bitwise AND2 : simulink/Logic and Bit Operations/Bitwise Operator  logicop=AND  UseBitMask=on  BitMask=bin2dec('00000000000000001111111100000000')  BitMaskRealWorld=Stored Integer
  Bitwise AND3 : simulink/Logic and Bit Operations/Bitwise Operator  logicop=AND  UseBitMask=on  BitMask=bin2dec('00000000111111110000000000000000')  BitMaskRealWorld=Stored Integer
  Bitwise AND4 : simulink/Logic and Bit Operations/Bitwise Operator  logicop=AND  UseBitMask=on  BitMask=bin2dec('11111111000000000000000000000000')  BitMaskRealWorld=Stored Integer
  Data Type Conversion{1,3..5} (4 alike) : DataTypeConversion  OutDataTypeStr=uint8
  Data Type Conversion2 : DataTypeConversion  OutDataTypeStr=uint32
  Mux2 : Mux
  Shift Arithmetic39 : ArithShift  BitShiftNumber=8  BitShiftDirection=Right
  Shift Arithmetic40 : ArithShift  BitShiftNumber=16  BitShiftDirection=Right
  Shift Arithmetic41 : ArithShift  BitShiftNumber=24  BitShiftDirection=Right
  Out1 : Outport
  wires:
  Data Type Conversion1/1 -> Mux2/4
  Data Type Conversion4/1 -> Mux2/2
  Data Type Conversion5/1 -> Mux2/3
  Data Type Conversion2/1 -> Bitwise AND2/1, Bitwise AND1/1, Bitwise AND3/1, Bitwise AND4/1
  Bitwise AND2/1 -> Shift Arithmetic39/1
  Data Type Conversion3/1 -> Mux2/1
  Shift Arithmetic39/1 -> Data Type Conversion5/1
  Bitwise AND3/1 -> Shift Arithmetic40/1
  In1/1 -> Data Type Conversion2/1
  Mux2/1 -> Out1/1
  Shift Arithmetic41/1 -> Data Type Conversion3/1
  Shift Arithmetic40/1 -> Data Type Conversion4/1
  Bitwise AND1/1 -> Data Type Conversion1/1
  Bitwise AND4/1 -> Shift Arithmetic41/1

== system SWC_HALOUT_type/run_SWC_HALOUT_Tx_5ms_sys/OUTP_AFTER/DID_list/uint32Touint8Array65 ==
  In1 : Inport
  Bitwise AND1 : simulink/Logic and Bit Operations/Bitwise Operator  logicop=AND  UseBitMask=on  BitMask=bin2dec('00000000000000000000000011111111')  BitMaskRealWorld=Stored Integer
  Bitwise AND2 : simulink/Logic and Bit Operations/Bitwise Operator  logicop=AND  UseBitMask=on  BitMask=bin2dec('00000000000000001111111100000000')  BitMaskRealWorld=Stored Integer
  Bitwise AND3 : simulink/Logic and Bit Operations/Bitwise Operator  logicop=AND  UseBitMask=on  BitMask=bin2dec('00000000111111110000000000000000')  BitMaskRealWorld=Stored Integer
  Bitwise AND4 : simulink/Logic and Bit Operations/Bitwise Operator  logicop=AND  UseBitMask=on  BitMask=bin2dec('11111111000000000000000000000000')  BitMaskRealWorld=Stored Integer
  Data Type Conversion{1,3..5} (4 alike) : DataTypeConversion  OutDataTypeStr=uint8
  Data Type Conversion2 : DataTypeConversion  OutDataTypeStr=uint32
  Mux2 : Mux
  Shift Arithmetic39 : ArithShift  BitShiftNumber=8  BitShiftDirection=Right
  Shift Arithmetic40 : ArithShift  BitShiftNumber=16  BitShiftDirection=Right
  Shift Arithmetic41 : ArithShift  BitShiftNumber=24  BitShiftDirection=Right
  Out1 : Outport
  wires:
  Data Type Conversion1/1 -> Mux2/4
  Data Type Conversion4/1 -> Mux2/2
  Data Type Conversion5/1 -> Mux2/3
  Data Type Conversion2/1 -> Bitwise AND2/1, Bitwise AND1/1, Bitwise AND3/1, Bitwise AND4/1
  Bitwise AND2/1 -> Shift Arithmetic39/1
  Data Type Conversion3/1 -> Mux2/1
  Shift Arithmetic39/1 -> Data Type Conversion5/1
  Bitwise AND3/1 -> Shift Arithmetic40/1
  In1/1 -> Data Type Conversion2/1
  Mux2/1 -> Out1/1
  Shift Arithmetic41/1 -> Data Type Conversion3/1
  Shift Arithmetic40/1 -> Data Type Conversion4/1
  Bitwise AND1/1 -> Data Type Conversion1/1
  Bitwise AND4/1 -> Shift Arithmetic41/1

== system SWC_HALOUT_type/run_SWC_HALOUT_Tx_5ms_sys/OUTP_AFTER/DID_list/uint32Touint8Array66 ==
  In1 : Inport
  Bitwise AND1 : simulink/Logic and Bit Operations/Bitwise Operator  logicop=AND  UseBitMask=on  BitMask=bin2dec('00000000000000000000000011111111')  BitMaskRealWorld=Stored Integer
  Bitwise AND2 : simulink/Logic and Bit Operations/Bitwise Operator  logicop=AND  UseBitMask=on  BitMask=bin2dec('00000000000000001111111100000000')  BitMaskRealWorld=Stored Integer
  Bitwise AND3 : simulink/Logic and Bit Operations/Bitwise Operator  logicop=AND  UseBitMask=on  BitMask=bin2dec('00000000111111110000000000000000')  BitMaskRealWorld=Stored Integer
  Bitwise AND4 : simulink/Logic and Bit Operations/Bitwise Operator  logicop=AND  UseBitMask=on  BitMask=bin2dec('11111111000000000000000000000000')  BitMaskRealWorld=Stored Integer
  Data Type Conversion{1,3..5} (4 alike) : DataTypeConversion  OutDataTypeStr=uint8
  Data Type Conversion2 : DataTypeConversion  OutDataTypeStr=uint32
  Mux2 : Mux
  Shift Arithmetic39 : ArithShift  BitShiftNumber=8  BitShiftDirection=Right
  Shift Arithmetic40 : ArithShift  BitShiftNumber=16  BitShiftDirection=Right
  Shift Arithmetic41 : ArithShift  BitShiftNumber=24  BitShiftDirection=Right
  Out1 : Outport
  wires:
  Bitwise AND4/1 -> Shift Arithmetic41/1
  Bitwise AND1/1 -> Data Type Conversion1/1
  Shift Arithmetic40/1 -> Data Type Conversion4/1
  Shift Arithmetic41/1 -> Data Type Conversion3/1
  Mux2/1 -> Out1/1
  In1/1 -> Data Type Conversion2/1
  Bitwise AND3/1 -> Shift Arithmetic40/1
  Shift Arithmetic39/1 -> Data Type Conversion5/1
  Data Type Conversion3/1 -> Mux2/1
  Bitwise AND2/1 -> Shift Arithmetic39/1
  Data Type Conversion2/1 -> Bitwise AND4/1, Bitwise AND3/1, Bitwise AND1/1, Bitwise AND2/1
  Data Type Conversion5/1 -> Mux2/3
  Data Type Conversion4/1 -> Mux2/2
  Data Type Conversion1/1 -> Mux2/4

== system SWC_HALOUT_type/run_SWC_HALOUT_Tx_5ms_sys/OUTP_AFTER/DID_list/uint32Touint8Array67 ==
  In1 : Inport
  Bitwise AND1 : simulink/Logic and Bit Operations/Bitwise Operator  logicop=AND  UseBitMask=on  BitMask=bin2dec('00000000000000000000000011111111')  BitMaskRealWorld=Stored Integer
  Bitwise AND2 : simulink/Logic and Bit Operations/Bitwise Operator  logicop=AND  UseBitMask=on  BitMask=bin2dec('00000000000000001111111100000000')  BitMaskRealWorld=Stored Integer
  Bitwise AND3 : simulink/Logic and Bit Operations/Bitwise Operator  logicop=AND  UseBitMask=on  BitMask=bin2dec('00000000111111110000000000000000')  BitMaskRealWorld=Stored Integer
  Bitwise AND4 : simulink/Logic and Bit Operations/Bitwise Operator  logicop=AND  UseBitMask=on  BitMask=bin2dec('11111111000000000000000000000000')  BitMaskRealWorld=Stored Integer
  Data Type Conversion{1,3..5} (4 alike) : DataTypeConversion  OutDataTypeStr=uint8
  Data Type Conversion2 : DataTypeConversion  OutDataTypeStr=uint32
  Mux2 : Mux
  Shift Arithmetic39 : ArithShift  BitShiftNumber=8  BitShiftDirection=Right
  Shift Arithmetic40 : ArithShift  BitShiftNumber=16  BitShiftDirection=Right
  Shift Arithmetic41 : ArithShift  BitShiftNumber=24  BitShiftDirection=Right
  Out1 : Outport
  wires:
  Data Type Conversion1/1 -> Mux2/4
  Data Type Conversion4/1 -> Mux2/2
  Data Type Conversion5/1 -> Mux2/3
  Data Type Conversion2/1 -> Bitwise AND2/1, Bitwise AND1/1, Bitwise AND3/1, Bitwise AND4/1
  Bitwise AND2/1 -> Shift Arithmetic39/1
  Data Type Conversion3/1 -> Mux2/1
  Shift Arithmetic39/1 -> Data Type Conversion5/1
  Bitwise AND3/1 -> Shift Arithmetic40/1
  In1/1 -> Data Type Conversion2/1
  Mux2/1 -> Out1/1
  Shift Arithmetic41/1 -> Data Type Conversion3/1
  Shift Arithmetic40/1 -> Data Type Conversion4/1
  Bitwise AND1/1 -> Data Type Conversion1/1
  Bitwise AND4/1 -> Shift Arithmetic41/1

== system SWC_HALOUT_type/run_SWC_HALOUT_Tx_5ms_sys/OUTP_AFTER/DID_list/uint32Touint8Array68 ==
  In1 : Inport
  Bitwise AND1 : simulink/Logic and Bit Operations/Bitwise Operator  logicop=AND  UseBitMask=on  BitMask=bin2dec('00000000000000000000000011111111')  BitMaskRealWorld=Stored Integer
  Bitwise AND2 : simulink/Logic and Bit Operations/Bitwise Operator  logicop=AND  UseBitMask=on  BitMask=bin2dec('00000000000000001111111100000000')  BitMaskRealWorld=Stored Integer
  Bitwise AND3 : simulink/Logic and Bit Operations/Bitwise Operator  logicop=AND  UseBitMask=on  BitMask=bin2dec('00000000111111110000000000000000')  BitMaskRealWorld=Stored Integer
  Bitwise AND4 : simulink/Logic and Bit Operations/Bitwise Operator  logicop=AND  UseBitMask=on  BitMask=bin2dec('11111111000000000000000000000000')  BitMaskRealWorld=Stored Integer
  Data Type Conversion{1,3..5} (4 alike) : DataTypeConversion  OutDataTypeStr=uint8
  Data Type Conversion2 : DataTypeConversion  OutDataTypeStr=uint32
  Mux2 : Mux
  Shift Arithmetic39 : ArithShift  BitShiftNumber=8  BitShiftDirection=Right
  Shift Arithmetic40 : ArithShift  BitShiftNumber=16  BitShiftDirection=Right
  Shift Arithmetic41 : ArithShift  BitShiftNumber=24  BitShiftDirection=Right
  Out1 : Outport
  wires:
  Bitwise AND4/1 -> Shift Arithmetic41/1
  Bitwise AND1/1 -> Data Type Conversion1/1
  Shift Arithmetic40/1 -> Data Type Conversion4/1
  Shift Arithmetic41/1 -> Data Type Conversion3/1
  Mux2/1 -> Out1/1
  In1/1 -> Data Type Conversion2/1
  Bitwise AND3/1 -> Shift Arithmetic40/1
  Shift Arithmetic39/1 -> Data Type Conversion5/1
  Data Type Conversion3/1 -> Mux2/1
  Bitwise AND2/1 -> Shift Arithmetic39/1
  Data Type Conversion2/1 -> Bitwise AND4/1, Bitwise AND3/1, Bitwise AND1/1, Bitwise AND2/1
  Data Type Conversion5/1 -> Mux2/3
  Data Type Conversion4/1 -> Mux2/2
  Data Type Conversion1/1 -> Mux2/4

== system SWC_HALOUT_type/run_SWC_HALOUT_Tx_5ms_sys/OUTP_AFTER/DID_list/uint32Touint8Array69 ==
  In1 : Inport
  Bitwise AND1 : simulink/Logic and Bit Operations/Bitwise Operator  logicop=AND  UseBitMask=on  BitMask=bin2dec('00000000000000000000000011111111')  BitMaskRealWorld=Stored Integer
  Bitwise AND2 : simulink/Logic and Bit Operations/Bitwise Operator  logicop=AND  UseBitMask=on  BitMask=bin2dec('00000000000000001111111100000000')  BitMaskRealWorld=Stored Integer
  Bitwise AND3 : simulink/Logic and Bit Operations/Bitwise Operator  logicop=AND  UseBitMask=on  BitMask=bin2dec('00000000111111110000000000000000')  BitMaskRealWorld=Stored Integer
  Bitwise AND4 : simulink/Logic and Bit Operations/Bitwise Operator  logicop=AND  UseBitMask=on  BitMask=bin2dec('11111111000000000000000000000000')  BitMaskRealWorld=Stored Integer
  Data Type Conversion{1,3..5} (4 alike) : DataTypeConversion  OutDataTypeStr=uint8
  Data Type Conversion2 : DataTypeConversion  OutDataTypeStr=uint32
  Mux2 : Mux
  Shift Arithmetic39 : ArithShift  BitShiftNumber=8  BitShiftDirection=Right
  Shift Arithmetic40 : ArithShift  BitShiftNumber=16  BitShiftDirection=Right
  Shift Arithmetic41 : ArithShift  BitShiftNumber=24  BitShiftDirection=Right
  Out1 : Outport
  wires:
  Bitwise AND4/1 -> Shift Arithmetic41/1
  Bitwise AND1/1 -> Data Type Conversion1/1
  Shift Arithmetic40/1 -> Data Type Conversion4/1
  Shift Arithmetic41/1 -> Data Type Conversion3/1
  Mux2/1 -> Out1/1
  In1/1 -> Data Type Conversion2/1
  Bitwise AND3/1 -> Shift Arithmetic40/1
  Shift Arithmetic39/1 -> Data Type Conversion5/1
  Data Type Conversion3/1 -> Mux2/1
  Bitwise AND2/1 -> Shift Arithmetic39/1
  Data Type Conversion2/1 -> Bitwise AND4/1, Bitwise AND3/1, Bitwise AND1/1, Bitwise AND2/1
  Data Type Conversion5/1 -> Mux2/3
  Data Type Conversion4/1 -> Mux2/2
  Data Type Conversion1/1 -> Mux2/4

== system SWC_HALOUT_type/run_SWC_HALOUT_Tx_5ms_sys/OUTP_AFTER/DID_list/uint32Touint8Array7 ==
  In1 : Inport
  Bitwise AND1 : simulink/Logic and Bit Operations/Bitwise Operator  logicop=AND  UseBitMask=on  BitMask=bin2dec('00000000000000000000000011111111')  BitMaskRealWorld=Stored Integer
  Bitwise AND2 : simulink/Logic and Bit Operations/Bitwise Operator  logicop=AND  UseBitMask=on  BitMask=bin2dec('00000000000000001111111100000000')  BitMaskRealWorld=Stored Integer
  Bitwise AND3 : simulink/Logic and Bit Operations/Bitwise Operator  logicop=AND  UseBitMask=on  BitMask=bin2dec('00000000111111110000000000000000')  BitMaskRealWorld=Stored Integer
  Bitwise AND4 : simulink/Logic and Bit Operations/Bitwise Operator  logicop=AND  UseBitMask=on  BitMask=bin2dec('11111111000000000000000000000000')  BitMaskRealWorld=Stored Integer
  Data Type Conversion{1,3..5} (4 alike) : DataTypeConversion  OutDataTypeStr=uint8
  Data Type Conversion2 : DataTypeConversion  OutDataTypeStr=uint32
  Mux2 : Mux
  Shift Arithmetic39 : ArithShift  BitShiftNumber=8  BitShiftDirection=Right
  Shift Arithmetic40 : ArithShift  BitShiftNumber=16  BitShiftDirection=Right
  Shift Arithmetic41 : ArithShift  BitShiftNumber=24  BitShiftDirection=Right
  Out1 : Outport
  wires:
  Data Type Conversion1/1 -> Mux2/4
  Data Type Conversion4/1 -> Mux2/2
  Data Type Conversion5/1 -> Mux2/3
  Data Type Conversion2/1 -> Bitwise AND2/1, Bitwise AND1/1, Bitwise AND3/1, Bitwise AND4/1
  Bitwise AND2/1 -> Shift Arithmetic39/1
  Data Type Conversion3/1 -> Mux2/1
  Shift Arithmetic39/1 -> Data Type Conversion5/1
  Bitwise AND3/1 -> Shift Arithmetic40/1
  In1/1 -> Data Type Conversion2/1
  Mux2/1 -> Out1/1
  Shift Arithmetic41/1 -> Data Type Conversion3/1
  Shift Arithmetic40/1 -> Data Type Conversion4/1
  Bitwise AND1/1 -> Data Type Conversion1/1
  Bitwise AND4/1 -> Shift Arithmetic41/1

== system SWC_HALOUT_type/run_SWC_HALOUT_Tx_5ms_sys/OUTP_AFTER/DID_list/uint32Touint8Array70 ==
  In1 : Inport
  Bitwise AND1 : simulink/Logic and Bit Operations/Bitwise Operator  logicop=AND  UseBitMask=on  BitMask=bin2dec('00000000000000000000000011111111')  BitMaskRealWorld=Stored Integer
  Bitwise AND2 : simulink/Logic and Bit Operations/Bitwise Operator  logicop=AND  UseBitMask=on  BitMask=bin2dec('00000000000000001111111100000000')  BitMaskRealWorld=Stored Integer
  Bitwise AND3 : simulink/Logic and Bit Operations/Bitwise Operator  logicop=AND  UseBitMask=on  BitMask=bin2dec('00000000111111110000000000000000')  BitMaskRealWorld=Stored Integer
  Bitwise AND4 : simulink/Logic and Bit Operations/Bitwise Operator  logicop=AND  UseBitMask=on  BitMask=bin2dec('11111111000000000000000000000000')  BitMaskRealWorld=Stored Integer
  Data Type Conversion{1,3..5} (4 alike) : DataTypeConversion  OutDataTypeStr=uint8
  Data Type Conversion2 : DataTypeConversion  OutDataTypeStr=uint32
  Mux2 : Mux
  Shift Arithmetic39 : ArithShift  BitShiftNumber=8  BitShiftDirection=Right
  Shift Arithmetic40 : ArithShift  BitShiftNumber=16  BitShiftDirection=Right
  Shift Arithmetic41 : ArithShift  BitShiftNumber=24  BitShiftDirection=Right
  Out1 : Outport
  wires:
  Data Type Conversion1/1 -> Mux2/4
  Data Type Conversion4/1 -> Mux2/2
  Data Type Conversion5/1 -> Mux2/3
  Data Type Conversion2/1 -> Bitwise AND2/1, Bitwise AND1/1, Bitwise AND3/1, Bitwise AND4/1
  Bitwise AND2/1 -> Shift Arithmetic39/1
  Data Type Conversion3/1 -> Mux2/1
  Shift Arithmetic39/1 -> Data Type Conversion5/1
  Bitwise AND3/1 -> Shift Arithmetic40/1
  In1/1 -> Data Type Conversion2/1
  Mux2/1 -> Out1/1
  Shift Arithmetic41/1 -> Data Type Conversion3/1
  Shift Arithmetic40/1 -> Data Type Conversion4/1
  Bitwise AND1/1 -> Data Type Conversion1/1
  Bitwise AND4/1 -> Shift Arithmetic41/1
